simulink library "determinePhase"  (R2016b)
settings: Solver=VariableStepAuto  StartTime=0.0  StopTime=10.0  RelTol=1e-3
undefined symbols (not defined in the file or in its folder): sitDownHip, standUpHip, stepSwingLegHip, StepType
settings Model: Creator=Nathan  LastModifiedBy=snyke7

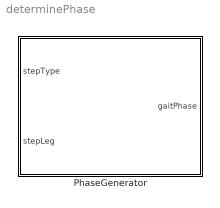
== system determinePhase ==
  PhaseGenerator : Subsystem

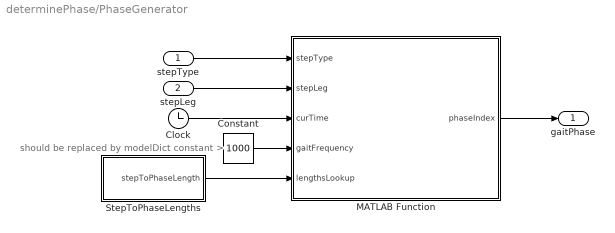
== system determinePhase/PhaseGenerator ==
  note: should be replaced by modelDict constant >
  stepType : Inport
  stepLeg : Inport  Port=2
  Clock : Clock
  Constant : Constant  Value=1000
  MATLAB Function : MATLAB Function  TreatAsAtomicUnit=on
  StepToPhaseLengths : Subsystem
  gaitPhase : Outport
  wires:
  MATLAB Function/1(phaseIndex) -> gaitPhase/1
  stepType/1 -> MATLAB Function/1(stepType)
  stepLeg/1 -> MATLAB Function/2(stepLeg)
  Clock/1 -> MATLAB Function/3(curTime)
  Constant/1 -> MATLAB Function/4(gaitFrequency)
  StepToPhaseLengths/1(stepToPhaseLength) -> MATLAB Function/5(lengthsLookup)

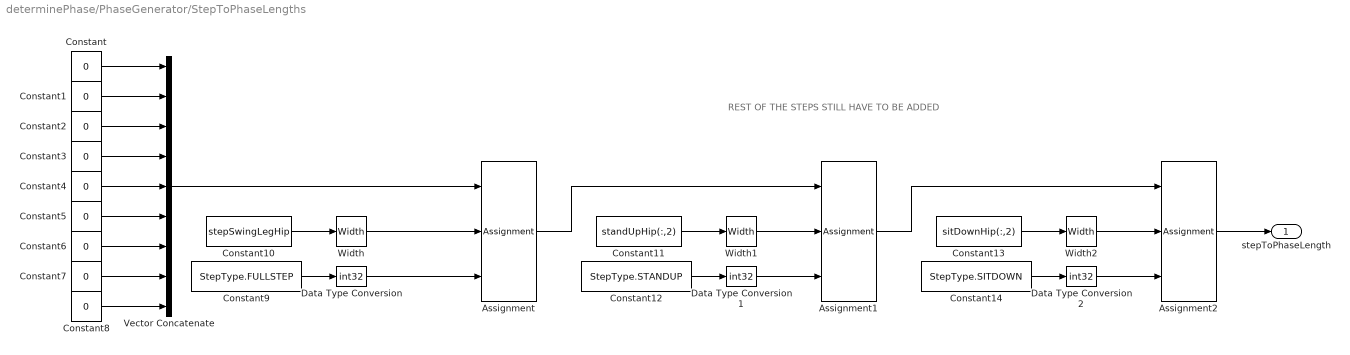
== system determinePhase/PhaseGenerator/StepToPhaseLengths ==
  note: REST OF THE STEPS STILL HAVE TO BE ADDED
  Assignment : Assignment  DiagnosticForDimensions=Warning  IndexOptions=Index vector (port)  Indices=1  OutputSizes=1
  Assignment1 : Assignment  DiagnosticForDimensions=Warning  IndexOptions=Index vector (port)  Indices=1  OutputSizes=1
  Assignment2 : Assignment  DiagnosticForDimensions=Warning  IndexOptions=Index vector (port)  Indices=1  OutputSizes=1
  Constant{,1..8} (9 alike) : Constant  Value=0
  Constant10 : Constant  Value=stepSwingLegHip
  Constant11 : Constant  Value=standUpHip(:,2)
  Constant12 : Constant  Value=StepType.STANDUP
  Constant13 : Constant  Value=sitDownHip(:,2)
  Constant14 : Constant  Value=StepType.SITDOWN
  Constant9 : Constant  Value=StepType.FULLSTEP
  Data Type Conversion : DataTypeConversion  OutDataTypeStr=int32
  Data Type Conversion1 : DataTypeConversion  OutDataTypeStr=int32
  Data Type Conversion2 : DataTypeConversion  OutDataTypeStr=int32
  Vector Concatenate : Concatenate  NumInputs=9
  Width : Width
  Width1 : Width
  Width2 : Width
  stepToPhaseLength : Outport
  wires:
  Constant2/1 -> Vector Concatenate/3
  Constant/1 -> Vector Concatenate/1
  Constant1/1 -> Vector Concatenate/2
  Constant3/1 -> Vector Concatenate/4
  Constant4/1 -> Vector Concatenate/5
  Constant5/1 -> Vector Concatenate/6
  Constant6/1 -> Vector Concatenate/7
  Constant7/1 -> Vector Concatenate/8
  Constant8/1 -> Vector Concatenate/9
  Vector Concatenate/1 -> Assignment/1
  Constant9/1 -> Data Type Conversion/1
  Data Type Conversion/1 -> Assignment/3
  Width/1 -> Assignment/2
  Constant10/1 -> Width/1
  Assignment/1 -> Assignment1/1
  Constant12/1 -> Data Type Conversion1/1
  Data Type Conversion1/1 -> Assignment1/3
  Width1/1 -> Assignment1/2
  Constant11/1 -> Width1/1
  Assignment1/1 -> Assignment2/1
  Constant14/1 -> Data Type Conversion2/1
  Data Type Conversion2/1 -> Assignment2/3
  Width2/1 -> Assignment2/2
  Constant13/1 -> Width2/1
  Assignment2/1 -> stepToPhaseLength/1

== matlab function determinePhase/PhaseGenerator/MATLAB Function ==
  data: stepType input; phaseIndex output; stepLeg input; curTime input; gaitFrequency input; lengthsLookup input
function phaseIndex   = getGaitPhases(stepType, stepLeg, curTime, gaitFrequency, lengthsLookup)
% wrapper for getGaitPhases
phaseIndex = getGaitPhases(stepType, stepLeg, curTime, gaitFrequency, lengthsLookup);
end
